simulink model "MarutiSwiftDesirepoweredby50HP240VDC"  (R2024b)
settings: Solver=VariableStepAuto  StartTime=0.0  StopTime=200  RelTol=1e-3
libraries: spsDCMachineLib x1, simulink x1, spsControlledVoltageSourceLib x1, spsDCVoltageSourceLib x1, sps_lib x1
settings Model: Creator=brain  LastModifiedBy=brain

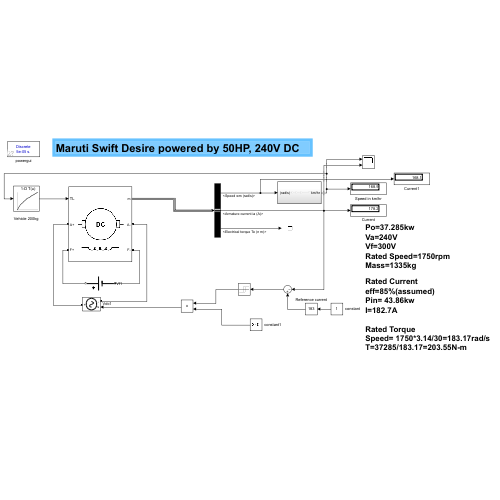
[thumbnail: Simulink's stored preview of the top-level diagram]
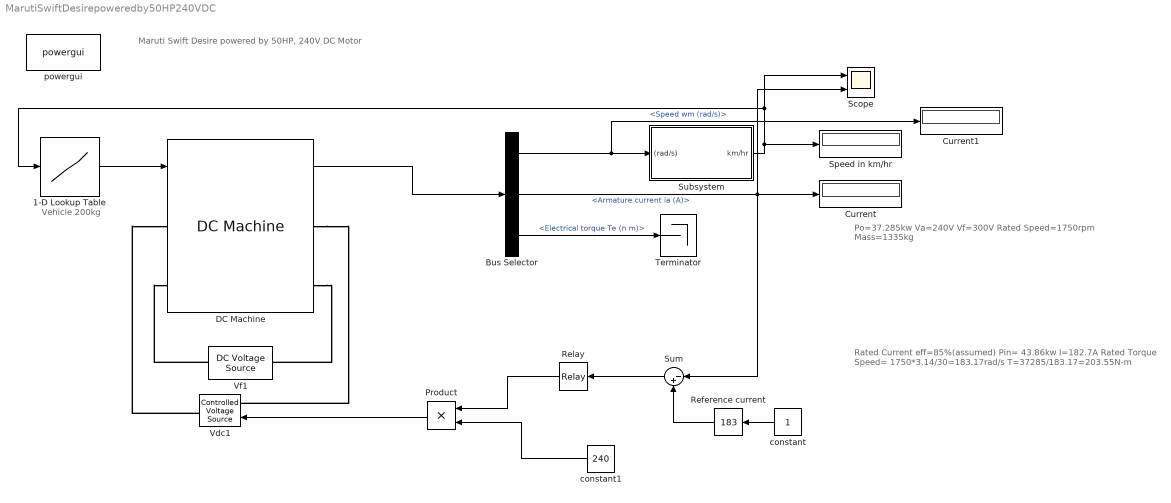
== system MarutiSwiftDesirepoweredby50HP240VDC ==
  note: Rated Current
      | eff=85%(assumed)
      | Pin= 43.86kw
      | I=182.7A
      |
      | Rated Torque
      | Speed= 1750*3.14/30=183.17rad/s
      | T=37285/183.17=203.55N-m
  note: Po=37.285kw
      | Va=240V
      | Vf=300V
      | Rated Speed=1750rpm
      | Mass=1335kg
  note: Maruti Swift Desire powered by 50HP, 240V DC Motor
  note: Vehicle 200kg
  1-D Lookup Table : Lookup_n-D  NumberOfTableDimensions=1  BreakpointsForDimension1=[5 10 15 20 25 30 35 40 45 50 55 60 65 70 75 80 85 90 95 100]  Table=[28.4 40.16 49.19 56.8 63.5 69.56 75.13 80.32 85.19 89.8 94.19 98.37 102.4 106.3 110 113.6 117.1 120.5 123.8 127]  InternalRulePriority=Speed  RndMeth=Simplest
  Bus Selector : BusSelector  OutputSignals=Speed wm (rad/s),Armature current ia (A),Electrical torque Te (n m)
  Current : Display
  Current1 : Display
  DC Machine : spsDCMachineLib/DC Machine  PresetModel=No  MechanicalLoad=Torque TL  FieldType=Wound  ShowDetailedParameters=on  MeasurementBus=off  RLa="[ 0.13  0.001558]"  RLf="[ 84.91  13.39]"  Laf=0.3406  MachineConstant=Torque constant (N.m/A)  Ke=1.8  Kt=1.8  J=1335*0.279*0.279  Bm=0.007032  Tf=5.282  w0=1  Ifinit=3.53315274997056  TsPowergui=0  TsBlock=-1
  Product : Product
  Reference current : simulink/Math Operations/Slider Gain  gain=183  low=1  high=187
  Relay : Relay  OnSwitchValue=2  OffSwitchValue=-2
  Scope : Scope  NumInputPorts=2
  Speed in km/hr : Display
  Subsystem : Subsystem
  Sum : Sum  Inputs=|-+
  Terminator : Terminator
  Vdc1 : spsControlledVoltageSourceLib/Controlled Voltage Source  Initialize=on  Source_Type=DC  Amplitude=0  Phase=0  Frequency=0  Measurements=None
  Vf1 : spsDCVoltageSourceLib/DC Voltage Source  Amplitude=300  Measurements=None
  constant : Constant
  constant1 : Constant  Value=240
  powergui : sps_lib/powergui  Priority=1  SimulationMode=Discrete  SampleTime=50e-6  frequency=60  Iterations=50  frequencyindice=0  Pbase=100e6  ErrMax=1e-4  UnitsV=kV  UnitsW=MW  buscounter=0  FunctionMessages=off  echomessages=off  EnableUseOfTLC=off  CurrentSourceSwitches=off  DisableSnubberDevices=off  DisableRonSwitches=off  DisableVfSwitches=off  DisplayEquations=off  AutomaticDiscreteSolvers=off  SolverType=Tustin/Backward Euler (TBE)  Interpol=off  ExternalGateDelay=off  methode=off  Ts=100  x0status=blocks  SPID=on  SwTol=0  HookPort=off  NonlinearTolerance=1e-4  nMaxIteration=100  ContinueOnMaxIteration=off  RestoreLinks=warning  ResistiveCurrentMeasurement=off  Frange=[0:2:500]  Ylog=off  Xlog=on  ShowGrid=off  save=off  variable=ZData  structure=0  ZoomFFT=off  StartTime=0.0  cycles=1  DisplayStyle=1  fundamental=60  FreqAxis=off  MaxFrequency=1000  frequencyindicesteady=1  RmsSteady=1  display=off
  wires:
  Bus Selector/1 -> Current1/1, Subsystem/1(" (rad/s)")  "<Speed wm (rad/s)>"
  Subsystem/1(km/hr) -> Scope/1, 1-D Lookup Table/1, Speed in km/hr/1
  1-D Lookup Table/1 -> DC Machine/1
  DC Machine/1 -> Bus Selector/1
  Bus Selector/3 -> Terminator/1  "<Electrical torque Te (n m)>"
  Bus Selector/2 -> Scope/2, Sum/1, Current/1  "<Armature current ia (A)>"
  Reference current/1 -> Sum/2
  Product/1 -> Vdc1/1
  Relay/1 -> Product/1
  constant1/1 -> Product/2
  constant/1 -> Reference current/1
  Sum/1 -> Relay/1
  connections:
  DC Machine/RConn1 -- Vdc1/LConn1
  Vf1/RConn1 -- DC Machine/LConn2
  Vdc1/RConn1 -- DC Machine/LConn1
  DC Machine/RConn2 -- Vf1/LConn1

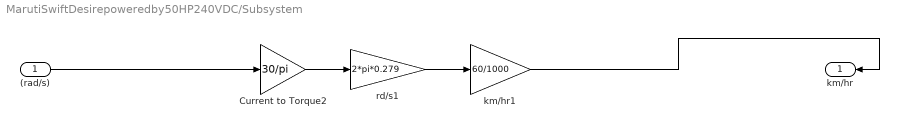
== system MarutiSwiftDesirepoweredby50HP240VDC/Subsystem ==
  " (rad/s)" : Inport
  Current to Torque2 : Gain  Gain=30/pi
  km/hr1 : Gain  Gain=60/1000
  rd/s1 : Gain  Gain=2*pi*0.279
  km/hr : Outport
  wires:
  " (rad/s)"/1 -> Current to Torque2/1
  Current to Torque2/1 -> rd/s1/1
  rd/s1/1 -> km/hr1/1
  km/hr1/1 -> km/hr/1
